simulink model "CM650A_HwTq0Meas"  (R2013b)
settings: Solver=FixedStepDiscrete  StartTime=0.0  StopTime=20  FixedStep=0.002  RelTol=1e-3
values from neighbouring files (symbols this model uses):
  ELECGLBPRM_HWTQOFFS_HWNWTMTR_F32 = DataDict.Constant    [CM650A_HwTq0Meas_DataDict.m]
  ELECGLBPRM_HWTQSATNLOWRLIM_HWNWTMTR_F32 = DataDict.Constant    [CM650A_HwTq0Meas_DataDict.m]
  ELECGLBPRM_HWTQSATNUPPRLIM_HWNWTMTR_F32 = DataDict.Constant    [CM650A_HwTq0Meas_DataDict.m]
  ELECGLBPRM_HWTQSCA_ULS_F32 = DataDict.Constant    [CM650A_HwTq0Meas_DataDict.m]
  ELECGLBPRM_NOFLT_CNT_U08 = DataDict.Constant    [CM650A_HwTq0Meas_DataDict.m]
  ELECGLBPRM_OFFSTRIMNOTPRFM_CNT_U08 = DataDict.Constant    [CM650A_HwTq0Meas_DataDict.m]
  ELECGLBPRM_PRTCLFLT_CNT_U08 = DataDict.Constant    [CM650A_HwTq0Meas_DataDict.m]
  ELECGLBPRM_SNSRINTFLT_CNT_U08 = DataDict.Constant    [CM650A_HwTq0Meas_DataDict.m]
  FLTINJ_HWTQ0MEAS_HWTQ0 = DataDict.Constant    [CM650A_HwTq0Meas_DataDict.m]
  FLTINJ_HWTQ0MEAS_TESTOK0 = DataDict.Constant    [CM650A_HwTq0Meas_DataDict.m]
  HwTq0MeasHwTq0PrtclFltFailStep = DataDict.Calibration    [CM650A_HwTq0Meas_DataDict.m]
  HwTq0MeasHwTq0PrtclFltPassStep = DataDict.Calibration    [CM650A_HwTq0Meas_DataDict.m]
  RACKLIMRCCWEOTSCA_ULS_F32 = DataDict.Constant    [CM650A_HwTq0Meas_DataDict.m]
  RACKLIMRCWEOTSCA_ULS_F32 = DataDict.Constant    [CM650A_HwTq0Meas_DataDict.m]
undefined symbols (not defined in the file or in its folder): NtcNr1, NtcSts1, sigbuilder_block, SigQlfr1
libraries: simulink x23, NxtrNvM x3, NxtrLim x2
(part 3 of 3)

== system CM650A_HwTq0Meas/HwTq0Meas/HwTq0MeasPer1/PrtclFltEvln/NoNewMsg ==
  Action Port : ActionPort  ActionType=else
  Add : Sum
  Bus Creator : BusCreator  Inputs=3
  Constant1 : Constant  OutDataTypeStr=uint32
  CopyRight2 : Subsystem  Description=|  mask(Copyright Information){none=on}
      | Copyright info block.                                               
      |                                                                     
      | Place copyright information at the top of every subsystem in design.
      mask prompts: none "No parameters"
      mask help: Place copyright information at the top of every subsystem in design.
      mask Display:
      | NxtrConf = 'Nexteer Confidential';
      | 
      | sys = bdroot; %handle for the current model ("system")
      | first = get_param(sys,'Created');
      | first = first(end-3:end);  %year is last four digits
      | 
      | last = get_param(sys,'LastModifiedDate');
      | if isempty(last)
      |     last = datestr(now,'yyyy');
      | else
      |     last = last(end-3:end);
      | end
      | 
      | if strcmp(first,last)
      |     fprintf('%s -- Copyright %s Nexteer',NxtrConf,first)
      | else
      |     fprintf('%s -- %s%s- %s Nexteer',NxtrConf,char(169),first,last)
      | end
  Data Type Conversion : DataTypeConversion  OutDataTypeStr=uint8
  NtcSts : simulink/Sources/Enumerated Constant  OutDataTypeStr=Enum: NtcSts1  Value=NtcSts1.NTCSTS_PREFAILD  SampleTime=inf
  PIM : DataStoreWrite  RequirementInfo={} %GIDa_f291a3bc_583c_4145_ae72_75310625072d  DataStoreName=HwTq0MsgMissRxCnt
  PIM1 : DataStoreRead  DataStoreName=HwTq0MsgMissRxCnt
  PRTCL_FAULT : Constant  Value=ELECGLBPRM_PRTCLFLT_CNT_U08  OutDataTypeStr=uint8
  Signal Conversion : SignalConversion
  Trq : Constant  Value=0  OutDataTypeStr=uint32
  Out1 : Outport
  wires:
  NtcSts/1 -> Data Type Conversion/1
  PRTCL_FAULT/1 -> Bus Creator/3  "ParamByte"
  Data Type Conversion/1 -> Bus Creator/2  "TestOk"
  Trq/1 -> Bus Creator/1  "RawHwTq"
  Bus Creator/1 -> Signal Conversion/1
  Signal Conversion/1 -> Out1/1
  Add/1 -> PIM/1
  Constant1/1 -> Add/2
  PIM1/1 -> Add/1

== system CM650A_HwTq0Meas/HwTq0Meas/HwTq0MeasPer1/RackLimrEot/CopyRight2 ==

== system CM650A_HwTq0Meas/HwTq0Meas/HwTq0MeasPer1/RackLimrEot/DoNothing ==
  Action Port : ActionPort  ActionType=else
  CopyRight2 : Subsystem  Description=|  mask(Copyright Information){none=on}
      | Copyright info block.                                               
      |                                                                     
      | Place copyright information at the top of every subsystem in design.
      mask prompts: none "No parameters"
      mask help: Place copyright information at the top of every subsystem in design.
      mask Display:
      | NxtrConf = 'Nexteer Confidential';
      | 
      | sys = bdroot; %handle for the current model ("system")
      | first = get_param(sys,'Created');
      | first = first(end-3:end);  %year is last four digits
      | 
      | last = get_param(sys,'LastModifiedDate');
      | if isempty(last)
      |     last = datestr(now,'yyyy');
      | else
      |     last = last(end-3:end);
      | end
      | 
      | if strcmp(first,last)
      |     fprintf('%s -- Copyright %s Nexteer',NxtrConf,first)
      | else
      |     fprintf('%s -- %s%s- %s Nexteer',NxtrConf,char(169),first,last)
      | end

== system CM650A_HwTq0Meas/HwTq0Meas/HwTq0MeasPer1/RackLimrEot/RackLimrEotSigRead2 ==
  RackLimrEotSig0SND : Inport
  RackLimrEotSig0CS : Inport  Port=2
  RackLimrEotSig0MsgID : Inport  Port=3
  RackLimrEotSig0MsgData : Inport  Port=4
  Action Port : ActionPort  ActionType=then
  CopyRight2 : Subsystem  Description=|  mask(Copyright Information){none=on}
      | Copyright info block.                                               
      |                                                                     
      | Place copyright information at the top of every subsystem in design.
      mask prompts: none "No parameters"
      mask help: Place copyright information at the top of every subsystem in design.
      mask Display:
      | NxtrConf = 'Nexteer Confidential';
      | 
      | sys = bdroot; %handle for the current model ("system")
      | first = get_param(sys,'Created');
      | first = first(end-3:end);  %year is last four digits
      | 
      | last = get_param(sys,'LastModifiedDate');
      | if isempty(last)
      |     last = datestr(now,'yyyy');
      | else
      |     last = last(end-3:end);
      | end
      | 
      | if strcmp(first,last)
      |     fprintf('%s -- Copyright %s Nexteer',NxtrConf,first)
      | else
      |     fprintf('%s -- %s%s- %s Nexteer',NxtrConf,char(169),first,last)
      | end
  DoNothing : Subsystem  TreatAsAtomicUnit=on
  If2 : If  NumInputs=2  IfExpression=(u1 ~= 0)&(u2==0)
  RackLimrEotSigRead1 : Subsystem  RequirementInfo={} %GIDa_7549db0e_b9f9_45da_b7a0_93b08f17cae8  TreatAsAtomicUnit=on
  wires:
  If2/1 -> RackLimrEotSigRead1/Action
  If2/2 -> DoNothing/Action
  RackLimrEotSig0CS/1 -> If2/2
  RackLimrEotSig0MsgID/1 -> RackLimrEotSigRead1/1(RackLimrEotSig0MsgID)
  RackLimrEotSig0SND/1 -> If2/1
  RackLimrEotSig0MsgData/1 -> RackLimrEotSigRead1/2(RackLimrEotSig0MsgData)

== system CM650A_HwTq0Meas/HwTq0Meas/HwTq0MeasPer1/Read the Flag/CopyRight2 ==

== system CM650A_HwTq0Meas/HwTq0Meas/HwTq0MeasPer1/SetNtcSts/CopyRight2 ==

== system CM650A_HwTq0Meas/HwTq0Meas/HwTq0MeasPer2/If Action Subsystem/CopyRight2 ==

== system CM650A_HwTq0Meas/HwTq0Meas/HwTq0MeasPer2/If Action Subsystem1/CopyRight2 ==

== system CM650A_HwTq0Meas/HwTq0Meas/HwTq0MeasPer2/SetNtcSts/CopyRight2 ==

== system CM650A_HwTq0Meas/HwTq0Meas/HwTq0MeasTrigStrt/GetRefTmr1MicroSec32bit/CopyRight2 ==

== system CM650A_HwTq0Meas/HwTq0Meas/HwTq0MeasTrigStrt/GetTiSpan1MicroSec32bit/CopyRight2 ==

== system CM650A_HwTq0Meas/HwTq0Meas/HwTq0MeasPer1/PrtclFltEvln/NewMsg/CopyRight2 ==

== system CM650A_HwTq0Meas/HwTq0Meas/HwTq0MeasPer1/PrtclFltEvln/NewMsg/FltInj_u08 ==
  note: Inport #2 must be constant
      | Const: FltInjectionLocType
  note: EA4.x Fault Injection
  note: This block requires no modification by FDD author.
      |
      | This block does not actually simulate any fault injection.  It is simply a pass-thru.
      |
      | The Const port (#2) simply terminates its signal, but we are trying to force the FDD author
      | to properly use the FltInjectionLocType enumeration in FDD model.
  Signal : Inport
  Const : Inport  Port=2
  Terminator : Terminator
  Out1 : Outport
  wires:
  Const/1 -> Terminator/1
  Signal/1 -> Out1/1

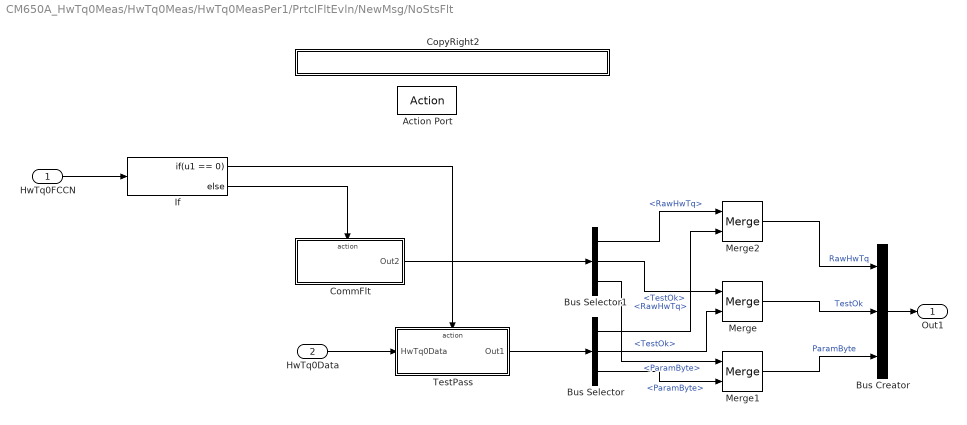
== system CM650A_HwTq0Meas/HwTq0Meas/HwTq0MeasPer1/PrtclFltEvln/NewMsg/NoStsFlt ==
  HwTq0FCCN : Inport
  HwTq0Data : Inport  Port=2
  Action Port : ActionPort  ActionType=then
  Bus Creator : BusCreator  Inputs=3
  Bus Selector : BusSelector  OutputSignals=RawHwTq,TestOk,ParamByte
  Bus Selector1 : BusSelector  OutputSignals=RawHwTq,TestOk,ParamByte
  CommFlt : Subsystem  RequirementInfo={'linktype_rmi_doors' '0000c468 (/ESG Group/FDD Module Requirements/EA4 Specific/CM650A_HwTq0Meas)' '#CM650A_23' 'true' 'REQ: CM650A_23' '' ; 'linktype_rmi_doors' '0000c468 (/ESG Group/FDD Module Requirements/EA4 Specific/CM650A_HwTq0Meas)' '#CM650A_48' 'true' 'REQ: CM650A_48' '' } %GIDa_a181911d_9433_49e5_ad17_4bc594fa1b0c  TreatAsAtomicUnit=on
      mask Display: disp('CommFlt')
  CopyRight2 : Subsystem  Description=|  mask(Copyright Information){none=on}
      | Copyright info block.                                               
      |                                                                     
      | Place copyright information at the top of every subsystem in design.
      mask prompts: none "No parameters"
      mask help: Place copyright information at the top of every subsystem in design.
      mask Display:
      | NxtrConf = 'Nexteer Confidential';
      | 
      | sys = bdroot; %handle for the current model ("system")
      | first = get_param(sys,'Created');
      | first = first(end-3:end);  %year is last four digits
      | 
      | last = get_param(sys,'LastModifiedDate');
      | if isempty(last)
      |     last = datestr(now,'yyyy');
      | else
      |     last = last(end-3:end);
      | end
      | 
      | if strcmp(first,last)
      |     fprintf('%s -- Copyright %s Nexteer',NxtrConf,first)
      | else
      |     fprintf('%s -- %s%s- %s Nexteer',NxtrConf,char(169),first,last)
      | end
  If : If  IfExpression=u1 == 0
  Merge : Merge
  Merge1 : Merge
  Merge2 : Merge
  TestPass : Subsystem  RequirementInfo={'linktype_rmi_doors' '0000c468 (/ESG Group/FDD Module Requirements/EA4 Specific/CM650A_HwTq0Meas)' '#CM650A_47' 'true' 'REQ: CM650A_47' '' } %GIDa_eb2d61f5_a171_4ae7_8550_49e90430938b  TreatAsAtomicUnit=on
      mask Display: disp('TESTPASS')
  Out1 : Outport
  wires:
  HwTq0FCCN/1 -> If/1
  If/1 -> TestPass/Action
  If/2 -> CommFlt/Action
  Merge/1 -> Bus Creator/2  "TestOk"
  Merge1/1 -> Bus Creator/3  "ParamByte"
  Merge2/1 -> Bus Creator/1  "RawHwTq"
  TestPass/1(Out1) -> Bus Selector/1
  CommFlt/1(Out2) -> Bus Selector1/1
  Bus Selector1/1 -> Merge2/1  "<RawHwTq>"
  Bus Selector/1 -> Merge2/2  "<RawHwTq>"
  Bus Selector1/2 -> Merge/1  "<TestOk>"
  Bus Selector1/3 -> Merge1/1  "<ParamByte>"
  Bus Selector/2 -> Merge/2  "<TestOk>"
  Bus Selector/3 -> Merge1/2  "<ParamByte>"
  Bus Creator/1 -> Out1/1
  HwTq0Data/1 -> TestPass/1(HwTq0Data)

== system CM650A_HwTq0Meas/HwTq0Meas/HwTq0MeasPer1/PrtclFltEvln/NewMsg/StsFlt ==
  Action Port : ActionPort  ActionType=else
  Add : Sum
  Bus Creator : BusCreator  Inputs=3
  Constant : Constant  OutDataTypeStr=uint8
  CopyRight2 : Subsystem  Description=|  mask(Copyright Information){none=on}
      | Copyright info block.                                               
      |                                                                     
      | Place copyright information at the top of every subsystem in design.
      mask prompts: none "No parameters"
      mask help: Place copyright information at the top of every subsystem in design.
      mask Display:
      | NxtrConf = 'Nexteer Confidential';
      | 
      | sys = bdroot; %handle for the current model ("system")
      | first = get_param(sys,'Created');
      | first = first(end-3:end);  %year is last four digits
      | 
      | last = get_param(sys,'LastModifiedDate');
      | if isempty(last)
      |     last = datestr(now,'yyyy');
      | else
      |     last = last(end-3:end);
      | end
      | 
      | if strcmp(first,last)
      |     fprintf('%s -- Copyright %s Nexteer',NxtrConf,first)
      | else
      |     fprintf('%s -- %s%s- %s Nexteer',NxtrConf,char(169),first,last)
      | end
  Data Store Read : DataStoreRead  DataStoreName=HwTq0ComStsErrCntr
  Data Store Write : DataStoreWrite  DataStoreName=HwTq0ComStsErrCntr
  Data Type Conversion : DataTypeConversion  OutDataTypeStr=uint8
  HwTq : Constant  Value=0  OutDataTypeStr=uint32
  NtcSts : simulink/Sources/Enumerated Constant  OutDataTypeStr=Enum: NtcSts1  Value=NtcSts1.NTCSTS_PREFAILD  SampleTime=inf
  PRTCL_FAULT : Constant  Value=ELECGLBPRM_PRTCLFLT_CNT_U08  OutDataTypeStr=uint8
  Signal Conversion : SignalConversion
  Out1 : Outport
  wires:
  PRTCL_FAULT/1 -> Bus Creator/3  "ParamByte"
  NtcSts/1 -> Data Type Conversion/1
  HwTq/1 -> Bus Creator/1  "RawHwTq"
  Bus Creator/1 -> Signal Conversion/1
  Signal Conversion/1 -> Out1/1
  Data Type Conversion/1 -> Bus Creator/2  "TestOk"
  Data Store Read/1 -> Add/1
  Constant/1 -> Add/2
  Add/1 -> Data Store Write/1

== system CM650A_HwTq0Meas/HwTq0Meas/HwTq0MeasPer1/PrtclFltEvln/NoNewMsg/CopyRight2 ==

== system CM650A_HwTq0Meas/HwTq0Meas/HwTq0MeasPer1/RackLimrEot/DoNothing/CopyRight2 ==

== system CM650A_HwTq0Meas/HwTq0Meas/HwTq0MeasPer1/RackLimrEot/RackLimrEotSigRead2/CopyRight2 ==

== system CM650A_HwTq0Meas/HwTq0Meas/HwTq0MeasPer1/RackLimrEot/RackLimrEotSigRead2/DoNothing ==
  Action Port : ActionPort  ActionType=else
  CopyRight2 : Subsystem  Description=|  mask(Copyright Information){none=on}
      | Copyright info block.                                               
      |                                                                     
      | Place copyright information at the top of every subsystem in design.
      mask prompts: none "No parameters"
      mask help: Place copyright information at the top of every subsystem in design.
      mask Display:
      | NxtrConf = 'Nexteer Confidential';
      | 
      | sys = bdroot; %handle for the current model ("system")
      | first = get_param(sys,'Created');
      | first = first(end-3:end);  %year is last four digits
      | 
      | last = get_param(sys,'LastModifiedDate');
      | if isempty(last)
      |     last = datestr(now,'yyyy');
      | else
      |     last = last(end-3:end);
      | end
      | 
      | if strcmp(first,last)
      |     fprintf('%s -- Copyright %s Nexteer',NxtrConf,first)
      | else
      |     fprintf('%s -- %s%s- %s Nexteer',NxtrConf,char(169),first,last)
      | end

== system CM650A_HwTq0Meas/HwTq0Meas/HwTq0MeasPer1/RackLimrEot/RackLimrEotSigRead2/RackLimrEotSigRead1 ==
  RackLimrEotSig0MsgID : Inport
  RackLimrEotSig0MsgData : Inport  Port=2
  Action Port : ActionPort  ActionType=then
  CopyRight2 : Subsystem  Description=|  mask(Copyright Information){none=on}
      | Copyright info block.                                               
      |                                                                     
      | Place copyright information at the top of every subsystem in design.
      mask prompts: none "No parameters"
      mask help: Place copyright information at the top of every subsystem in design.
      mask Display:
      | NxtrConf = 'Nexteer Confidential';
      | 
      | sys = bdroot; %handle for the current model ("system")
      | first = get_param(sys,'Created');
      | first = first(end-3:end);  %year is last four digits
      | 
      | last = get_param(sys,'LastModifiedDate');
      | if isempty(last)
      |     last = datestr(now,'yyyy');
      | else
      |     last = last(end-3:end);
      | end
      | 
      | if strcmp(first,last)
      |     fprintf('%s -- Copyright %s Nexteer',NxtrConf,first)
      | else
      |     fprintf('%s -- %s%s- %s Nexteer',NxtrConf,char(169),first,last)
      | end
  EotDataPending : Subsystem  RequirementInfo={} %GIDa_a13e0620_73b5_4e5b_9869_65330fe2c72c  TreatAsAtomicUnit=on
  EotDataReceived : Subsystem  RequirementInfo={'linktype_rmi_doors' '0000c468 (/ESG Group/FDD Module Requirements/EA4 Specific/CM650A_HwTq0Meas)' '#CM650A_68' 'true' 'REQ: CM650A_68' '' ; 'linktype_rmi_doors' '0000c468 (/ESG Group/FDD Module Requirements/EA4 Specific/CM650A_HwTq0Meas)' '#CM650A_69' 'true' 'REQ: CM650A_69' '' } %GIDa_bfc73ea9_52f7_4540_ba60_4a9740f9a96a  TreatAsAtomicUnit=on
  If : If  NumInputs=3  IfExpression=(u1==1)&(u2==1)&(u3==1)
  PIM : DataStoreRead  DataStoreName=RackLimrEot0Id2DataReadCmpl
  PIM1 : DataStoreRead  DataStoreName=RackLimrEot0Id3DataReadCmpl
  PIM2 : DataStoreRead  DataStoreName=RackLimrEot0Id4DataReadCmpl
  wires:
  PIM/1 -> If/1
  If/2 -> EotDataPending/Action  "False"
  If/1 -> EotDataReceived/Action  "True"
  RackLimrEotSig0MsgID/1 -> EotDataPending/1(RackLimrEotSig0MsgID)
  PIM1/1 -> If/2
  PIM2/1 -> If/3
  RackLimrEotSig0MsgData/1 -> EotDataPending/2(RackLimrEotSig0MsgData)

== system CM650A_HwTq0Meas/HwTq0Meas/HwTq0MeasPer1/PrtclFltEvln/NewMsg/NoStsFlt/CommFlt ==
  Action Port : ActionPort  ActionType=else
  Add : Sum
  Bus Creator1 : BusCreator  Inputs=3
  Constant : Constant  OutDataTypeStr=uint8
  CopyRight2 : Subsystem  Description=|  mask(Copyright Information){none=on}
      | Copyright info block.                                               
      |                                                                     
      | Place copyright information at the top of every subsystem in design.
      mask prompts: none "No parameters"
      mask help: Place copyright information at the top of every subsystem in design.
      mask Display:
      | NxtrConf = 'Nexteer Confidential';
      | 
      | sys = bdroot; %handle for the current model ("system")
      | first = get_param(sys,'Created');
      | first = first(end-3:end);  %year is last four digits
      | 
      | last = get_param(sys,'LastModifiedDate');
      | if isempty(last)
      |     last = datestr(now,'yyyy');
      | else
      |     last = last(end-3:end);
      | end
      | 
      | if strcmp(first,last)
      |     fprintf('%s -- Copyright %s Nexteer',NxtrConf,first)
      | else
      |     fprintf('%s -- %s%s- %s Nexteer',NxtrConf,char(169),first,last)
      | end
  Data Store Read : DataStoreRead  DataStoreName=HwTq0IntSnsrErrCntr
  Data Store Write : DataStoreWrite  DataStoreName=HwTq0IntSnsrErrCntr
  Data Type Conversion : DataTypeConversion  OutDataTypeStr=uint8
  Flt : Constant  Value=ELECGLBPRM_SNSRINTFLT_CNT_U08  OutDataTypeStr=uint8
  HwTq : Constant  Value=0  OutDataTypeStr=uint32
  NtcSts : simulink/Sources/Enumerated Constant  OutDataTypeStr=Enum: NtcSts1  Value=NtcSts1.NTCSTS_PREFAILD  SampleTime=inf
  Signal Conversion1 : SignalConversion
  Out2 : Outport
  wires:
  Flt/1 -> Bus Creator1/3  "ParamByte"
  NtcSts/1 -> Data Type Conversion/1
  HwTq/1 -> Bus Creator1/1  "RawHwTq"
  Bus Creator1/1 -> Signal Conversion1/1
  Signal Conversion1/1 -> Out2/1
  Data Type Conversion/1 -> Bus Creator1/2  "TestOk"
  Data Store Read/1 -> Add/1
  Constant/1 -> Add/2
  Add/1 -> Data Store Write/1

== system CM650A_HwTq0Meas/HwTq0Meas/HwTq0MeasPer1/PrtclFltEvln/NewMsg/NoStsFlt/CopyRight2 ==

== system CM650A_HwTq0Meas/HwTq0Meas/HwTq0MeasPer1/PrtclFltEvln/NewMsg/NoStsFlt/TestPass ==
  HwTq0Data : Inport
  Action Port : ActionPort  ActionType=then
  Bus Creator : BusCreator  Inputs=3
  CopyRight2 : Subsystem  Description=|  mask(Copyright Information){none=on}
      | Copyright info block.                                               
      |                                                                     
      | Place copyright information at the top of every subsystem in design.
      mask prompts: none "No parameters"
      mask help: Place copyright information at the top of every subsystem in design.
      mask Display:
      | NxtrConf = 'Nexteer Confidential';
      | 
      | sys = bdroot; %handle for the current model ("system")
      | first = get_param(sys,'Created');
      | first = first(end-3:end);  %year is last four digits
      | 
      | last = get_param(sys,'LastModifiedDate');
      | if isempty(last)
      |     last = datestr(now,'yyyy');
      | else
      |     last = last(end-3:end);
      | end
      | 
      | if strcmp(first,last)
      |     fprintf('%s -- Copyright %s Nexteer',NxtrConf,first)
      | else
      |     fprintf('%s -- %s%s- %s Nexteer',NxtrConf,char(169),first,last)
      | end
  Data Type Conversion : DataTypeConversion  OutDataTypeStr=uint8
  NoFlt : Constant  RequirementInfo={} %GIDa_e64df96d_f0ef_4edd_b9a4_9c46566b9362  Value=ELECGLBPRM_NOFLT_CNT_U08  OutDataTypeStr=uint8
  NtcSts1 : simulink/Sources/Enumerated Constant  OutDataTypeStr=Enum: NtcSts1  Value=NtcSts1.NTCSTS_PREPASSD  SampleTime=inf
  Signal Conversion : SignalConversion
  Out1 : Outport
  wires:
  NtcSts1/1 -> Data Type Conversion/1
  Data Type Conversion/1 -> Bus Creator/2  "TestOk"
  NoFlt/1 -> Bus Creator/3  "ParamByte"
  HwTq0Data/1 -> Bus Creator/1  "RawHwTq"
  Bus Creator/1 -> Signal Conversion/1
  Signal Conversion/1 -> Out1/1

== system CM650A_HwTq0Meas/HwTq0Meas/HwTq0MeasPer1/PrtclFltEvln/NewMsg/StsFlt/CopyRight2 ==

== system CM650A_HwTq0Meas/HwTq0Meas/HwTq0MeasPer1/RackLimrEot/RackLimrEotSigRead2/DoNothing/CopyRight2 ==

== system CM650A_HwTq0Meas/HwTq0Meas/HwTq0MeasPer1/RackLimrEot/RackLimrEotSigRead2/RackLimrEotSigRead1/CopyRight2 ==

== system CM650A_HwTq0Meas/HwTq0Meas/HwTq0MeasPer1/RackLimrEot/RackLimrEotSigRead2/RackLimrEotSigRead1/EotDataPending ==
  RackLimrEotSig0MsgID : Inport
  RackLimrEotSig0MsgData : Inport  Port=2
  Action Port : ActionPort  ActionType=else
  CopyRight2 : Subsystem  Description=|  mask(Copyright Information){none=on}
      | Copyright info block.                                               
      |                                                                     
      | Place copyright information at the top of every subsystem in design.
      mask prompts: none "No parameters"
      mask help: Place copyright information at the top of every subsystem in design.
      mask Display:
      | NxtrConf = 'Nexteer Confidential';
      | 
      | sys = bdroot; %handle for the current model ("system")
      | first = get_param(sys,'Created');
      | first = first(end-3:end);  %year is last four digits
      | 
      | last = get_param(sys,'LastModifiedDate');
      | if isempty(last)
      |     last = datestr(now,'yyyy');
      | else
      |     last = last(end-3:end);
      | end
      | 
      | if strcmp(first,last)
      |     fprintf('%s -- Copyright %s Nexteer',NxtrConf,first)
      | else
      |     fprintf('%s -- %s%s- %s Nexteer',NxtrConf,char(169),first,last)
      | end
  Donothing : Subsystem  TreatAsAtomicUnit=on
  Read2 : Subsystem  TreatAsAtomicUnit=on
  Read3 : Subsystem  TreatAsAtomicUnit=on
  Read4 : Subsystem  TreatAsAtomicUnit=on
  Switch Case : SwitchCase  CaseConditions={2,3,4}
  wires:
  RackLimrEotSig0MsgID/1 -> Switch Case/1
  Switch Case/4 -> Donothing/Action  "NoValidMsgId"
  Switch Case/1 -> Read2/Action
  Switch Case/2 -> Read3/Action
  Switch Case/3 -> Read4/Action
  RackLimrEotSig0MsgData/1 -> Read4/1(RackLimrEotSig0MsgData), Read3/1(RackLimrEotSig0MsgData), Read2/1(RackLimrEotSig0MsgData)

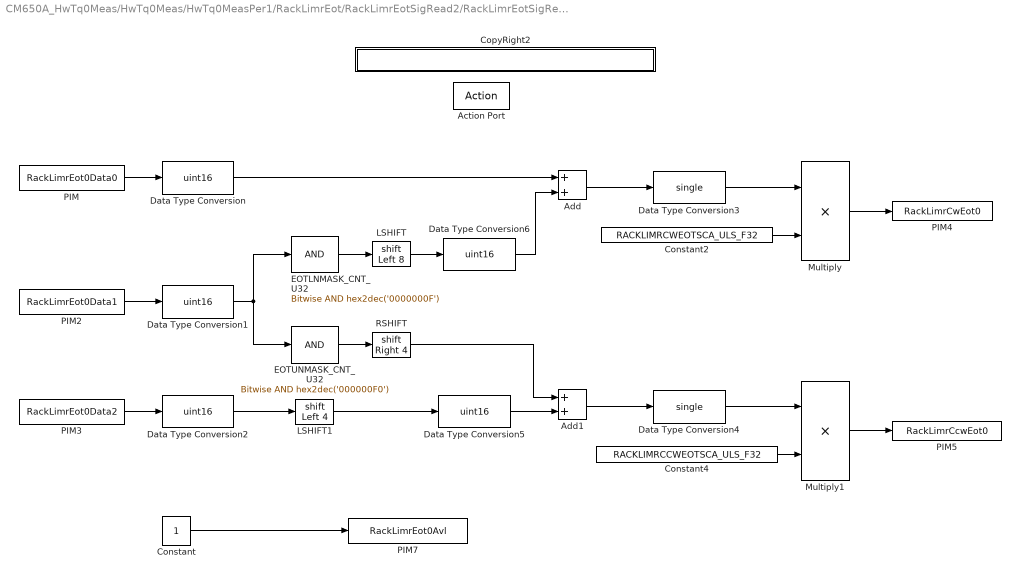
== system CM650A_HwTq0Meas/HwTq0Meas/HwTq0MeasPer1/RackLimrEot/RackLimrEotSigRead2/RackLimrEotSigRead1/EotDataReceived ==
  Action Port : ActionPort  ActionType=then
  Add : Sum
  Add1 : Sum
  Constant : Constant  OutDataTypeStr=boolean
  Constant2 : Constant  Value=RACKLIMRCWEOTSCA_ULS_F32
  Constant4 : Constant  Value=RACKLIMRCCWEOTSCA_ULS_F32
  CopyRight2 : Subsystem  Description=|  mask(Copyright Information){none=on}
      | Copyright info block.                                               
      |                                                                     
      | Place copyright information at the top of every subsystem in design.
      mask prompts: none "No parameters"
      mask help: Place copyright information at the top of every subsystem in design.
      mask Display:
      | NxtrConf = 'Nexteer Confidential';
      | 
      | sys = bdroot; %handle for the current model ("system")
      | first = get_param(sys,'Created');
      | first = first(end-3:end);  %year is last four digits
      | 
      | last = get_param(sys,'LastModifiedDate');
      | if isempty(last)
      |     last = datestr(now,'yyyy');
      | else
      |     last = last(end-3:end);
      | end
      | 
      | if strcmp(first,last)
      |     fprintf('%s -- Copyright %s Nexteer',NxtrConf,first)
      | else
      |     fprintf('%s -- %s%s- %s Nexteer',NxtrConf,char(169),first,last)
      | end
  Data Type Conversion{,1..2,5..6} (5 alike) : DataTypeConversion  OutDataTypeStr=uint16
  Data Type Conversion3 : DataTypeConversion  OutDataTypeStr=single
  Data Type Conversion4 : DataTypeConversion  OutDataTypeStr=single
  EOTLNMASK_CNT_U32 : simulink/Logic and Bit Operations/Bitwise Operator  logicop=AND  UseBitMask=on  BitMask=hex2dec('0000000F')  BitMaskRealWorld=Stored Integer
  EOTUNMASK_CNT_U32 : simulink/Logic and Bit Operations/Bitwise Operator  logicop=AND  UseBitMask=on  BitMask=hex2dec('000000F0')  BitMaskRealWorld=Stored Integer
  LSHIFT : ArithShift  BitShiftNumber=8  BitShiftDirection=Left
  LSHIFT1 : ArithShift  BitShiftNumber=4  BitShiftDirection=Left
  Multiply : Product  Inputs=**
  Multiply1 : Product  Inputs=**
  PIM : DataStoreRead  DataStoreName=RackLimrEot0Data0
  PIM2 : DataStoreRead  DataStoreName=RackLimrEot0Data1
  PIM3 : DataStoreRead  DataStoreName=RackLimrEot0Data2
  PIM4 : DataStoreWrite  DataStoreName=RackLimrCwEot0
  PIM5 : DataStoreWrite  DataStoreName=RackLimrCcwEot0
  PIM7 : DataStoreWrite  DataStoreName=RackLimrEot0Avl
  RSHIFT : ArithShift  BitShiftNumber=4  BitShiftDirection=Right
  wires:
  Constant/1 -> PIM7/1
  PIM/1 -> Data Type Conversion/1
  PIM2/1 -> Data Type Conversion1/1
  EOTLNMASK_CNT_U32/1 -> LSHIFT/1
  LSHIFT/1 -> Data Type Conversion6/1
  EOTUNMASK_CNT_U32/1 -> RSHIFT/1
  RSHIFT/1 -> Add1/1
  PIM3/1 -> Data Type Conversion2/1
  LSHIFT1/1 -> Data Type Conversion5/1
  Add/1 -> Data Type Conversion3/1
  Add1/1 -> Data Type Conversion4/1
  Multiply/1 -> PIM4/1
  Constant2/1 -> Multiply/2
  Constant4/1 -> Multiply1/2
  Multiply1/1 -> PIM5/1
  Data Type Conversion/1 -> Add/1
  Data Type Conversion1/1 -> EOTLNMASK_CNT_U32/1, EOTUNMASK_CNT_U32/1
  Data Type Conversion2/1 -> LSHIFT1/1
  Data Type Conversion3/1 -> Multiply/1
  Data Type Conversion4/1 -> Multiply1/1
  Data Type Conversion5/1 -> Add1/2
  Data Type Conversion6/1 -> Add/2

== system CM650A_HwTq0Meas/HwTq0Meas/HwTq0MeasPer1/PrtclFltEvln/NewMsg/NoStsFlt/CommFlt/CopyRight2 ==

== system CM650A_HwTq0Meas/HwTq0Meas/HwTq0MeasPer1/PrtclFltEvln/NewMsg/NoStsFlt/TestPass/CopyRight2 ==

== system CM650A_HwTq0Meas/HwTq0Meas/HwTq0MeasPer1/RackLimrEot/RackLimrEotSigRead2/RackLimrEotSigRead1/EotDataPending/CopyRight2 ==

== system CM650A_HwTq0Meas/HwTq0Meas/HwTq0MeasPer1/RackLimrEot/RackLimrEotSigRead2/RackLimrEotSigRead1/EotDataPending/Donothing ==
  Action Port : ActionPort  ActionType=default
  CopyRight2 : Subsystem  Description=|  mask(Copyright Information){none=on}
      | Copyright info block.                                               
      |                                                                     
      | Place copyright information at the top of every subsystem in design.
      mask prompts: none "No parameters"
      mask help: Place copyright information at the top of every subsystem in design.
      mask Display:
      | NxtrConf = 'Nexteer Confidential';
      | 
      | sys = bdroot; %handle for the current model ("system")
      | first = get_param(sys,'Created');
      | first = first(end-3:end);  %year is last four digits
      | 
      | last = get_param(sys,'LastModifiedDate');
      | if isempty(last)
      |     last = datestr(now,'yyyy');
      | else
      |     last = last(end-3:end);
      | end
      | 
      | if strcmp(first,last)
      |     fprintf('%s -- Copyright %s Nexteer',NxtrConf,first)
      | else
      |     fprintf('%s -- %s%s- %s Nexteer',NxtrConf,char(169),first,last)
      | end

== system CM650A_HwTq0Meas/HwTq0Meas/HwTq0MeasPer1/RackLimrEot/RackLimrEotSigRead2/RackLimrEotSigRead1/EotDataPending/Read2 ==
  RackLimrEotSig0MsgData : Inport
  Action Port : ActionPort  ActionType=case
  Constant : Constant  OutDataTypeStr=boolean
  CopyRight2 : Subsystem  Description=|  mask(Copyright Information){none=on}
      | Copyright info block.                                               
      |                                                                     
      | Place copyright information at the top of every subsystem in design.
      mask prompts: none "No parameters"
      mask help: Place copyright information at the top of every subsystem in design.
      mask Display:
      | NxtrConf = 'Nexteer Confidential';
      | 
      | sys = bdroot; %handle for the current model ("system")
      | first = get_param(sys,'Created');
      | first = first(end-3:end);  %year is last four digits
      | 
      | last = get_param(sys,'LastModifiedDate');
      | if isempty(last)
      |     last = datestr(now,'yyyy');
      | else
      |     last = last(end-3:end);
      | end
      | 
      | if strcmp(first,last)
      |     fprintf('%s -- Copyright %s Nexteer',NxtrConf,first)
      | else
      |     fprintf('%s -- %s%s- %s Nexteer',NxtrConf,char(169),first,last)
      | end
  Data0 : DataStoreWrite  DataStoreName=RackLimrEot0Data0
  Data1 : DataStoreWrite  DataStoreName=RackLimrEot0Id2DataReadCmpl
  wires:
  Constant/1 -> Data1/1
  RackLimrEotSig0MsgData/1 -> Data0/1

== system CM650A_HwTq0Meas/HwTq0Meas/HwTq0MeasPer1/RackLimrEot/RackLimrEotSigRead2/RackLimrEotSigRead1/EotDataPending/Read3 ==
  RackLimrEotSig0MsgData : Inport
  Action Port : ActionPort  ActionType=case
  Constant : Constant  OutDataTypeStr=boolean
  CopyRight2 : Subsystem  Description=|  mask(Copyright Information){none=on}
      | Copyright info block.                                               
      |                                                                     
      | Place copyright information at the top of every subsystem in design.
      mask prompts: none "No parameters"
      mask help: Place copyright information at the top of every subsystem in design.
      mask Display:
      | NxtrConf = 'Nexteer Confidential';
      | 
      | sys = bdroot; %handle for the current model ("system")
      | first = get_param(sys,'Created');
      | first = first(end-3:end);  %year is last four digits
      | 
      | last = get_param(sys,'LastModifiedDate');
      | if isempty(last)
      |     last = datestr(now,'yyyy');
      | else
      |     last = last(end-3:end);
      | end
      | 
      | if strcmp(first,last)
      |     fprintf('%s -- Copyright %s Nexteer',NxtrConf,first)
      | else
      |     fprintf('%s -- %s%s- %s Nexteer',NxtrConf,char(169),first,last)
      | end
  Data1 : DataStoreWrite  DataStoreName=RackLimrEot0Id3DataReadCmpl
  SPD1 : DataStoreWrite  DataStoreName=RackLimrEot0Data1
  wires:
  RackLimrEotSig0MsgData/1 -> SPD1/1
  Constant/1 -> Data1/1

== system CM650A_HwTq0Meas/HwTq0Meas/HwTq0MeasPer1/RackLimrEot/RackLimrEotSigRead2/RackLimrEotSigRead1/EotDataPending/Read4 ==
  RackLimrEotSig0MsgData : Inport
  Action Port : ActionPort  ActionType=case
  Constant : Constant  OutDataTypeStr=boolean
  CopyRight2 : Subsystem  Description=|  mask(Copyright Information){none=on}
      | Copyright info block.                                               
      |                                                                     
      | Place copyright information at the top of every subsystem in design.
      mask prompts: none "No parameters"
      mask help: Place copyright information at the top of every subsystem in design.
      mask Display:
      | NxtrConf = 'Nexteer Confidential';
      | 
      | sys = bdroot; %handle for the current model ("system")
      | first = get_param(sys,'Created');
      | first = first(end-3:end);  %year is last four digits
      | 
      | last = get_param(sys,'LastModifiedDate');
      | if isempty(last)
      |     last = datestr(now,'yyyy');
      | else
      |     last = last(end-3:end);
      | end
      | 
      | if strcmp(first,last)
      |     fprintf('%s -- Copyright %s Nexteer',NxtrConf,first)
      | else
      |     fprintf('%s -- %s%s- %s Nexteer',NxtrConf,char(169),first,last)
      | end
  Data1 : DataStoreWrite  DataStoreName=RackLimrEot0Id4DataReadCmpl
  PIM : DataStoreWrite  DataStoreName=RackLimrEot0Data2
  wires:
  RackLimrEotSig0MsgData/1 -> PIM/1
  Constant/1 -> Data1/1

== system CM650A_HwTq0Meas/HwTq0Meas/HwTq0MeasPer1/RackLimrEot/RackLimrEotSigRead2/RackLimrEotSigRead1/EotDataReceived/CopyRight2 ==

== system CM650A_HwTq0Meas/HwTq0Meas/HwTq0MeasPer1/RackLimrEot/RackLimrEotSigRead2/RackLimrEotSigRead1/EotDataPending/Donothing/CopyRight2 ==

== system CM650A_HwTq0Meas/HwTq0Meas/HwTq0MeasPer1/RackLimrEot/RackLimrEotSigRead2/RackLimrEotSigRead1/EotDataPending/Read2/CopyRight2 ==

== system CM650A_HwTq0Meas/HwTq0Meas/HwTq0MeasPer1/RackLimrEot/RackLimrEotSigRead2/RackLimrEotSigRead1/EotDataPending/Read3/CopyRight2 ==

== system CM650A_HwTq0Meas/HwTq0Meas/HwTq0MeasPer1/RackLimrEot/RackLimrEotSigRead2/RackLimrEotSigRead1/EotDataPending/Read4/CopyRight2 ==

== stateflow chart CM650A_HwTq0Meas/HwTq0Meas/HwTq0MeasPer2/SetNtcSts/ISO Fault Debounce Design ==
  settings: stateMachineType=MEALY_MACHINE
  note: NTCSTS_PASSD           (0)
      | NTCSTS_FAILD             (1)
      | NTCSTS_PREPASSD   (2)
      | NTCSTS_PREFAILD     (3)
      |
      | SIGQLFR_NORES        (0)
      | SIGQLFR_PASSD         (1)
      | SIGQLFR_FAILD           (2)
  note: Pass Loop
  note: Fail Loop
  note: 
  (default) -> (junction 89)
  (junction 89) -> (junction 95) [order 1] : [NtcSts ==3]
  (junction 89) -> (junction 93) [order 2] : [NtcSts ==2]
  (junction 89) -> (junction 141) [order 3] : [NtcSts ==1]
      | { ErrAcc = 32767;
      | Qualifier =2;
      |  }
  (junction 89) -> (junction 141) [order 4] : [NtcSts ==0]
      | { ErrAcc = -32768;
      | Qualifier=1;
      | }
  (junction 95) -> (junction 103) [order 2]
  (junction 95) -> (junction 111) [order 1] : [ErrAcc <=0]
      | {ErrAcc = DebStep;}
  (junction 93) -> (junction 123) [order 2] : {
      | ErrAcc = ErrAcc - DebStep;
      | }
  (junction 93) -> (junction 123) [order 1] : [(ErrAcc - DebStep) <= -32768]
      | { ErrAcc = -32768;
      | Qualifier=1;
      | }
  (junction 103) -> (junction 111) [order 1] : [(ErrAcc + DebStep) <32767]
      | {ErrAcc = ErrAcc + DebStep;}
  (junction 103) -> (junction 111) [order 2] : {ErrAcc = 32767;
      | Qualifier =2;}
  (junction 123) -> (junction 141)
  (junction 111) -> (junction 141)
  (junction 141) -> (junction 159) [order 2] : {ErrAcc = 0;
      | Qualifier =0;
      | }
  (junction 141) -> (junction 159) [order 1] : [SvcClr ==0]
  data: NtcSts input uint8; Qualifier output uint8; DebStep input uint16; ErrAcc local single; SvcClr input

== stateflow chart CM650A_HwTq0Meas/HwTq0Meas/HwTq0MeasPer1/SetNtcSts/ISO Fault Debounce Design ==
  settings: stateMachineType=MEALY_MACHINE
  note: NTCSTS_PASSD           (0)
      | NTCSTS_FAILD             (1)
      | NTCSTS_PREPASSD   (2)
      | NTCSTS_PREFAILD     (3)
      |
      | SIGQLFR_NORES        (0)
      | SIGQLFR_PASSD         (1)
      | SIGQLFR_FAILD           (2)
  note: Pass Loop
  note: Fail Loop
  note: 
  (default) -> (junction 89)
  (junction 89) -> (junction 95) [order 1] : [NtcSts ==3]
  (junction 89) -> (junction 93) [order 2] : [NtcSts ==2]
  (junction 89) -> (junction 141) [order 3] : [NtcSts ==1]
      | { ErrAcc = 32767;
      | Qualifier =2;
      |  }
  (junction 89) -> (junction 141) [order 4] : [NtcSts ==0]
      | { ErrAcc = -32768;
      | Qualifier=1;
      | }
  (junction 95) -> (junction 103) [order 2]
  (junction 95) -> (junction 111) [order 1] : [ErrAcc <=0]
      | {ErrAcc = DebStep;}
  (junction 93) -> (junction 123) [order 2] : {
      | ErrAcc = ErrAcc - DebStep;
      | }
  (junction 93) -> (junction 123) [order 1] : [(ErrAcc - DebStep) <= -32768]
      | { ErrAcc = -32768;
      | Qualifier=1;
      | }
  (junction 103) -> (junction 111) [order 1] : [(ErrAcc + DebStep) <32767]
      | {ErrAcc = ErrAcc + DebStep;}
  (junction 103) -> (junction 111) [order 2] : {ErrAcc = 32767;
      | Qualifier =2;}
  (junction 123) -> (junction 141)
  (junction 111) -> (junction 141)
  (junction 141) -> (junction 159) [order 2] : {ErrAcc = 0;
      | Qualifier =0;
      | }
  (junction 141) -> (junction 159) [order 1] : [SvcClr ==0]
  data: NtcSts input uint8; Qualifier output uint8; DebStep input uint16; ErrAcc local int16; SvcClr input

== matlab function CM650A_HwTq0Meas/Simulated_Input/FRXDATA2/RackLimrEotCal ==
  data: SensId input; Cw input; Ccw input; RsentIdd output
function RsentIdd  = RackLimrEot (SensId, Cw, Ccw )
%#eml 

persistent CwCal1;
persistent CcwCal1;

RsentIdd = uint32(0);

CwCal1 = uint32(single(5.11875)*single(Cw));
CcwCal1 = uint32(single(5.11875)*single(Ccw));

RawData0 = bitand(CwCal1,uint32(255));

RawData1a = bitand(CwCal1,uint32(3840));
RawData1b = bitshift(RawData1a,-8);
RawData1c = bitand(CcwCal1,uint32(15));
RawData1d = bitshift(RawData1c,4);
RawData1 = RawData1b + RawData1d;

RawData2a = bitand(CcwCal1,uint32(4080));
RawData2 = bitshift(RawData2a,-4);

if (SensId ==2)
    RsentIdd = uint32(bitshift(SensId,8)) + RawData0;
elseif (SensId ==3)
    RsentIdd = uint32(bitshift(SensId,8)) + RawData1; 
elseif (SensId ==4)
    RsentIdd = uint32(bitshift(SensId,8)) + RawData2;
end
%%

== stateflow chart CM650A_HwTq0Meas/HwTq0Meas/HwTq0MeasPer1/RollCnt1 ==
  settings: stateMachineType=MEALY_MACHINE
  (default) -> (junction 89) : {HwTq0RollgCntr = HwTq0PrevRollgCntr;}
  (junction 89) -> (junction 169) [order 1] : [ (TestOk ==2) ]
  (junction 89) -> (junction 93) [order 2]
  (junction 169) -> (junction 93) [order 2] : {HwTq0RollgCntr = 0;}
  (junction 169) -> (junction 93) [order 1] : [(HwTq0RollgCntr+1) <= 255]
      | {HwTq0RollgCntr = HwTq0RollgCntr + 1;}
  (junction 93) -> (junction 188)
  data: HwTq0RollgCntr output uint8; TestOk input uint8; HwTq0PrevRollgCntr input uint8
